simulink model "Rigid_Axle"  (R2022a)
settings: Solver=VariableStepAuto  StartTime=0.0  StopTime=10.0  RelTol=1e-3
libraries: simulink x1
settings Model: Creator=joser  LastModifiedBy=joser
settings ModelReferenceCC: EnableRefExpFcnMdlSchedulingChecks=off
settings RTWCC: Description=Generic Real-Time Target

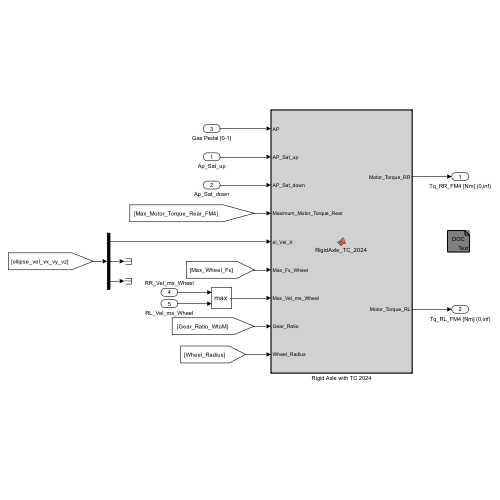
[thumbnail: Simulink's stored preview of the top-level diagram]
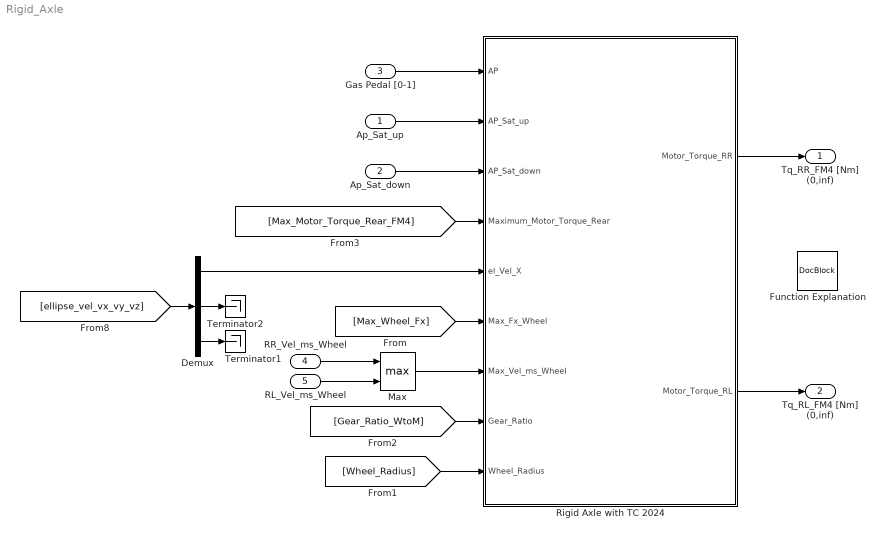
== system Rigid_Axle ==
  "Ap_Sat_up " : Inport
  Ap_Sat_down : Inport  Port=2
  Gas Pedal [0-1] : Inport  Port=3
  RR_Vel_ms_Wheel : Inport  Port=4
  RL_Vel_ms_Wheel : Inport  Port=5
  Demux : Demux  Outputs=3
  Function Explanation : simulink/Model-Wide Utilities/DocBlock  DocumentType=Text
      content=|
      | Comparing the speed of the Ellipse and the speed of the Wheels, we can
      | determine the % of deviation between both (which is the slip). With
      | calculations from the Tyres & Performance Department, we know that the
      | maximum optimal slip in a STRAIGHT line is 15%. Therefore (using the Magic
      | Formula), we can determine the maximum X-Force permissible by the Wheels
      | with that % of slip (which is the constant Max_Fx_Tyre, input
      | of Rigid Axle).
      |
      | With that and the radius of the Wheels, we can calculate the maximum
      | Torque for it to stop slipping.
  Max : MinMax  Function=max  Inputs=2
  "Rigid Axle with TC 2024 " : MATLAB Function  TreatAsAtomicUnit=on
  Terminator1 : Terminator
  Terminator2 : Terminator
  Tq_RR_FM4 [Nm] (0,inf) : Outport  VectorParamsAs1DForOutWhenUnconnected=off
  Tq_RL_FM4 [Nm] (0,inf) : Outport  Port=2  VectorParamsAs1DForOutWhenUnconnected=off
  wires:
  "Rigid Axle with TC 2024 "/1(Motor_Torque_RR) -> Tq_RR_FM4 [Nm] (0,inf)/1
  "Ap_Sat_up "/1 -> "Rigid Axle with TC 2024 "/2(AP_Sat_up)
  Gas Pedal [0-1]/1 -> "Rigid Axle with TC 2024 "/1(AP)
  "Rigid Axle with TC 2024 "/2(Motor_Torque_RL) -> Tq_RL_FM4 [Nm] (0,inf)/1
  Ap_Sat_down/1 -> "Rigid Axle with TC 2024 "/3(AP_Sat_down)
  [Max_Motor_Torque_Rear_FM4] -> "Rigid Axle with TC 2024 "/4(Maximum_Motor_Torque_Rear)
  [ellipse_vel_vx_vy_vz] -> Demux/1
  RR_Vel_ms_Wheel/1 -> Max/1
  RL_Vel_ms_Wheel/1 -> Max/2
  [Max_Wheel_Fx] -> "Rigid Axle with TC 2024 "/6(Max_Fx_Wheel)
  Demux/2 -> Terminator2/1
  Demux/3 -> Terminator1/1
  Demux/1 -> "Rigid Axle with TC 2024 "/5(el_Vel_X)
  Max/1 -> "Rigid Axle with TC 2024 "/7(Max_Vel_ms_Wheel)
  [Gear_Ratio_WtoM] -> "Rigid Axle with TC 2024 "/8(Gear_Ratio)
  [Wheel_Radius] -> "Rigid Axle with TC 2024 "/9(Wheel_Radius)

== matlab function Rigid_Axle/Rigid Axle with TC 2024  ==
  data: AP input; Motor_Torque_RR output; AP_Sat_up input; AP_Sat_down input; Maximum_Motor_Torque_Rear input; Motor_Torque_RL output; el_Vel_X input; Max_Fx_Wheel input; Max_Vel_ms_Wheel input; Gear_Ratio input; Wheel_Radius input
function [Motor_Torque_RR, Motor_Torque_RL] = RigidAxle_TC_2024(AP, AP_Sat_up, AP_Sat_down, Maximum_Motor_Torque_Rear, el_Vel_X, Max_Fx_Wheel, Max_Vel_ms_Wheel, Gear_Ratio, Wheel_Radius)

Slip = Max_Vel_ms_Wheel / el_Vel_X; % Percentage of slip
    %% Accelerator pedal with saturations

    if AP <= AP_Sat_down

        Throttle = 0; % If the real position of the pedal is lower than the minimum saturation --> lifted throttle.
        Pedal_pressed = 0;

    elseif AP >= AP_Sat_up

        Throttle = 1;  % If the real position of the pedal is higher than the maximum saturation --> full throttle.
        Pedal_pressed = 1;
    
    else
        Throttle = (AP - AP_Sat_down)/(AP_Sat_up - AP_Sat_down); % Compute the percentage of pedal pressed (if it is not 1 or 0) regarding the maximun and minimum saturation
        Pedal_pressed = 1;
    
    end

    %% Motor Torque

    if Slip < 1.15 % 15% of slip, greater than that number it is not optimal.

        Motor_Torque_RR = Maximum_Motor_Torque_Rear * Throttle; % Rear Right (RR) motor torque output.
        Motor_Torque_RL = Maximum_Motor_Torque_Rear * Throttle; % Rear Left (RL) motor torque output.
        % Percentage of Pedal = final percentage of Torque (referenced to Maximum_Torque_Rear).

    else 
        Motor_Torque_RR = Max_Fx_Wheel * Wheel_Radius * Gear_Ratio * Pedal_pressed; % Motor Torque RR output if tyre slips more than 15%.
        Motor_Torque_RL = Max_Fx_Wheel * Wheel_Radius * Gear_Ratio * Pedal_pressed; % Motor Torque RL output if tyre slips more than 15%.

        % EXPLANATION:
        % Max_Fx_Wheel * Wheel_Radius * Gear_Ratio = 
        % = Torque_Wheel * Gear_Ratio =
        % = Torque_Motor
        % Max_Fx_Tyre got it with Magic Formula MATLAB (Tyres & Performance guys) 
        % More information at the Doc outside the function.
        
    end
end
